simulink model "arm_angle_control_PID_with_hardware_model_protected_4"  (R2020b)
settings: Solver=FixedStepDiscrete  StartTime=0.0  StopTime=500  RelTol=1e-3
values from neighbouring files (symbols this model uses):
  ArmStartAngle = 89    [init.m]
  deltaT = 0.01    [init.m]
  FinalValue = -10    [init.m]
  InitialValue = 89    [init.m]
  StepTime = 200    [init.m]
libraries: pid_lib x1
settings Model: Creator=alpdemir  LastModifiedBy=emrecanacikgoz
settings SolverCC: AutoInsertRateTranBlk=on
settings DataIOCC: ReturnWorkspaceOutputs=off
settings DebuggingCC: ArithmeticOperatorsInVariantConditions=warning
settings SFSimCC: SimUseLocalCustomCode=off  CustomCodeUndefinedFunction=UseInterfaceOnly
settings RTWCC: RTWUseLocalCustomCode=off
settings CodeAppCC: StateflowObjectComments=on

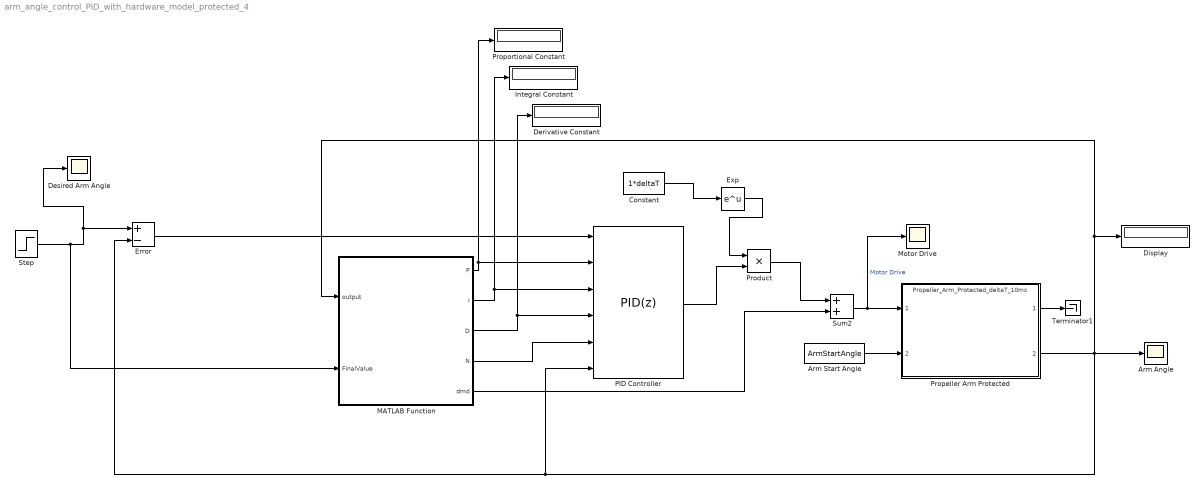
== system arm_angle_control_PID_with_hardware_model_protected_4 ==
  Arm Angle : Scope
  Arm Start Angle : Constant  Value=ArmStartAngle
  Constant : Constant  Value=1*deltaT
  Derivative Constant : Display
  Desired Arm Angle : Scope
  Display : Display
  Error : Sum  Inputs=+-
  Exp : Math  SaturateOnIntegerOverflow=on
  Integral Constant : Display
  MATLAB Function : MATLAB Function  TreatAsAtomicUnit=on
  Motor Drive : Scope
  PID Controller : pid_lib/PID Controller  Controller=PID  Form=Parallel  TimeDomain=Discrete-time  UseExternalTs=off  SampleTime=-1  IntegratorMethod=Forward Euler  FilterMethod=Forward Euler  ControllerParametersSource=external  P=1  I=0.1  D=0.5  UseFilter=on  N=100  TunerSelectOption=Transfer Function Based (PID Tuner App)  ZeroCross=off  InitialConditionSource=internal  InitialConditionForIntegrator=0  InitialConditionForFilter=0  DifferentiatorICPrevScaledInput=0  ExternalReset=rising  TrackingMode=off  Kt=1  LimitOutput=off  SatLimitsSource=internal  UpperSaturationLimit=inf  LowerSaturationLimit=-inf  LinearizeAsGain=off  AntiWindupMode=none  Kb=1  POutMin=[]  POutMax=[]  IOutMin=[]  IOutMax=[]  DOutMin=[]  DOutMax=[]  NOutMin=[]  NOutMax=[]  SumOutMin=[]  SumOutMax=[]  SaturationOutMin=[]  SaturationOutMax=[]  PParamMin=[]  PParamMax=[]  IParamMin=[]  IParamMax=[]  DParamMin=[]  DParamMax=[]  NParamMin=[]  NParamMax=[]  KbParamMin=[]  KbParamMax=[]  KtParamMin=[]  KtParamMax=[]  KbOutMin=[]  KbOutMax=[]  KtOutMin=[]  KtOutMax=[]  IntegratorOutMin=[]  IntegratorOutMax=[]  FilterOutMin=[]  FilterOutMax=[]  SumI1OutMin=[]  SumI1OutMax=[]  SumI2OutMin=[]  SumI2OutMax=[]  SumI3OutMin=[]  SumI3OutMax=[]  SumI4OutMin=[]  SumI4OutMax=[]  SumDOutMin=[]  SumDOutMax=[]  DifferentiatorOutMin=[]  DifferentiatorOutMax=[]  FilterDiffOutCoefMin=[]  FilterDiffOutCoefMax=[]  ReciprocalOutMin=[]  ReciprocalOutMax=[]  SumDenOutMin=[]  SumDenOutMax=[]  SumNumOutMin=[]  SumNumOutMax=[]  DivideOutMin=[]  DivideOutMax=[]  UdiffTsProdOutMin=[]  UdiffTsProdOutMax=[]  NTsProdOutMin=[]  NTsProdOutMax=[]  UintegralTsProdOutMin=[]  UintegralTsProdOutMax=[]  UngainTsProdOutMin=[]  UngainTsProdOutMax=[]  IntegratorContinuousStateAttributes=''  IntegratorStateMustResolveToSignalObject=off  IntegratorRTWStateStorageClass=Auto  FilterContinuousStateAttributes=''  FilterStateMustResolveToSignalObject=off  FilterRTWStateStorageClass=Auto  ParallelPVariant=ExternalParameters  IdealPVariant=Disabled  IVariant=ExternalParameters  DVariant=ExternalParameters  IntegratorVariant=Discrete  SatVariant=Disabled  AWVariant=Passthrough  PCopyVariant=Disabled  TRVariant=Disabled  FdbkBlocksVariant=Forward  IdealPFdbkVariant=Disabled  SatFdbkVariant=Disabled  DerivativeFilterVariant=ForwardEulerFilter  NVariant=ExternalParameters  NCopyVariant=Disabled  FilterICVariant=InternalICsFilter  IntegratorICVariant=InternalICs  ExternalResetVariant=ExternalReset  TRSumVariant=Passthrough  SumFdbkVariant=Disabled  SumVariant=Sum_PID  TsampFilterVariant=InternalTs  TsampNgainVariant=Passthrough  TsampIntegralVariant=Passthrough  ExternalSaturationOutDataTypeStr=Inherit: Same as second input
  Product : Product
  Propeller Arm Protected : ModelReference  ModelNameDialog=Propeller_Arm_Protected_deltaT_10ms.slxp  ModelReferenceVersion=3.39  CopyOfModelProtected=on
      mask Display: image('$imagefile'); % Use "Edit Image" on toolstrip to change.
  Proportional Constant : Display
  Step : Step  Time=StepTime  Before=InitialValue  After=FinalValue  SampleTime=deltaT
  Sum2 : Sum
  Terminator1 : Terminator
  wires:
  MATLAB Function/2(I) -> PID Controller/3, Integral Constant/1
  MATLAB Function/1(P) -> PID Controller/2, Proportional Constant/1
  MATLAB Function/3(D) -> Derivative Constant/1, PID Controller/4
  Sum2/1 -> Motor Drive/1, Propeller Arm Protected/1  "Motor Drive"
  Propeller Arm Protected/1 -> Terminator1/1
  Step/1 -> MATLAB Function/2(FinalValue), Desired Arm Angle/1, Error/1
  MATLAB Function/4(N) -> PID Controller/5
  Error/1 -> PID Controller/1
  Propeller Arm Protected/2 -> MATLAB Function/1(output), Display/1, PID Controller/6, Error/2, Arm Angle/1
  Arm Start Angle/1 -> Propeller Arm Protected/2
  MATLAB Function/5(dmd) -> Sum2/2
  Exp/1 -> Product/1
  Constant/1 -> Exp/1
  PID Controller/1 -> Product/2
  Product/1 -> Sum2/1

== matlab function arm_angle_control_PID_with_hardware_model_protected_4/MATLAB Function ==
  data: output input; P output; FinalValue input; I output; D output; N output; dmd output
function [P, I, D, N, dmd] = adaptive_parameters(output, FinalValue)
    if (FinalValue >= 75) && ((output >= 75) || ((30 >= output)&&(output > -20)) || ((75 > output)&&(output > 30)))
        P = 1.385;
        I = 0.01;
        D = 0.35;
        N = 53;
        dmd = 0;

    elseif ((15 >= FinalValue) && (FinalValue >= -20)) && (((30 >= output)&&(output > -20)) || ((47 >= output)&&(output > 30)))
        P = 2.445;
        I = 0.75;
        D = 1.5;
        N = 70;
        dmd = 40;

    elseif ((75 > FinalValue) && (FinalValue> 15)) && (((75 > output) && (output > 15)) || ((15 >= output)&&(output > -5)))
        P = 3;
        I = 1.75;
        D = 0.7;
        N = 100;
        dmd = 0;

    else
        P = 2.5;
        I = 0.1;
        D = 0.4;
        N = 100;
        dmd = 0;
    end
end
